simulink model "lab6_1"  (R2021a)
settings: Solver=VariableStepAuto  StartTime=0.0  StopTime=10.0  MaxStep=5e-4  RelTol=1e-3
settings Model: Creator=Luka  LastModifiedBy=Luka

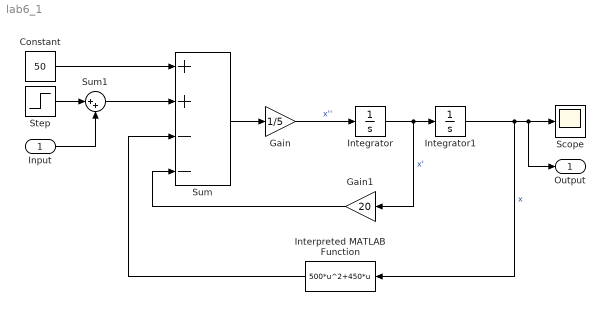
== system lab6_1 ==
  Input : Inport
  Constant : Constant  Value=50
  Gain : Gain  Gain=1/5
  Gain1 : Gain  Gain=20
  Integrator : Integrator
  Integrator1 : Integrator  InitialCondition=0.1
  Interpreted MATLAB Function : MATLABFcn  MATLABFcn=500*u^2+450*u
  Scope : Scope
  Step : Step  Time=5  SampleTime=0
  Sum : Sum  Inputs=++--
  Sum1 : Sum  Inputs=|++
  Output : Outport
  wires:
  Integrator/1 -> Gain1/1, Integrator1/1  "x'"
  Integrator1/1 -> Output/1, Scope/1, Interpreted MATLAB Function/1  "x"
  Gain/1 -> Integrator/1  "x''"
  Sum/1 -> Gain/1
  Constant/1 -> Sum/1
  Gain1/1 -> Sum/4
  Interpreted MATLAB Function/1 -> Sum/3
  Sum1/1 -> Sum/2
  Step/1 -> Sum1/1
  Input/1 -> Sum1/2
